simulink model "mdIGBTControlledCurrentSource"  (Simulink 7.3)
settings: Solver=ode45  StartTime=0.0  StopTime=0.5  RelTol=1e-3
libraries: powerlib x14
settings Model: Creator=Think79  LastModifiedBy=Think79

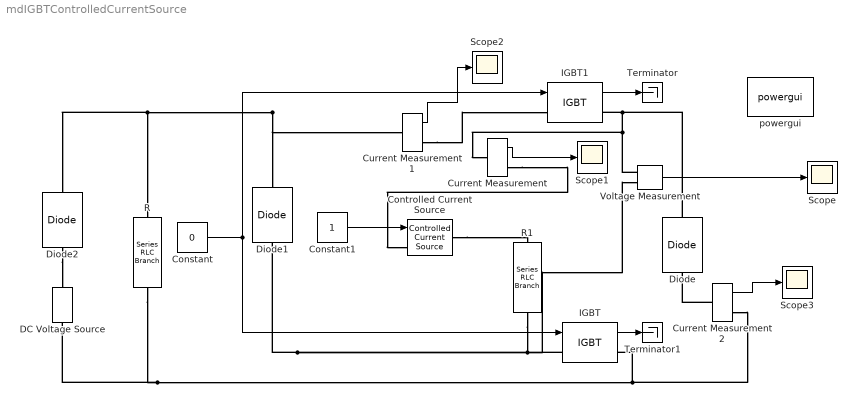
== system mdIGBTControlledCurrentSource ==
  Constant : Constant  Value=0  OutDataType=fixdt(1, 16)  OutScaling=2^0
  Constant1 : Constant  OutDataType=fixdt(1, 16)  OutScaling=2^0
  Controlled Current Source : powerlib/Electrical Sources/Controlled Current Source  DialogController=POWERSYS.PowerSysDialog  SystemSampleTime=-1  Initialize=on  Source_Type=AC  Amplitude=0  Phase=0  Frequency=0  Measurements=None
  Current Measurement : powerlib/Measurements/Current Measurement  DialogController=POWERSYS.PowerSysDialog  SystemSampleTime=-1  PhasorSimulation=off  OutputType=Complex  PSBequivalent=0
  Current Measurement1 : powerlib/Measurements/Current Measurement  DialogController=POWERSYS.PowerSysDialog  SystemSampleTime=-1  PhasorSimulation=off  OutputType=Complex  PSBequivalent=0
  Current Measurement2 : powerlib/Measurements/Current Measurement  DialogController=POWERSYS.PowerSysDialog  SystemSampleTime=-1  PhasorSimulation=off  OutputType=Complex  PSBequivalent=0
  DC Voltage Source : powerlib/Electrical Sources/DC Voltage Source  DialogController=POWERSYS.PowerSysDialog  SystemSampleTime=-1  Amplitude=60  Measurements=None
  Diode : powerlib/Power Electronics/Diode  DialogController=POWERSYS.PowerSysDialog  SystemSampleTime=-1  Ron=0.001  Lon=0  Vf=0.8  IC=0  UseSnubber=off  Rs=500  Cs=250e-9  Measurements=off
  Diode1 : powerlib/Power Electronics/Diode  DialogController=POWERSYS.PowerSysDialog  SystemSampleTime=-1  Ron=0.001  Lon=0  Vf=0.8  IC=0  UseSnubber=off  Rs=500  Cs=250e-9  Measurements=off
  Diode2 : powerlib/Power Electronics/Diode  DialogController=POWERSYS.PowerSysDialog  SystemSampleTime=-1  Ron=0.001  Lon=0  Vf=0.8  IC=0  UseSnubber=off  Rs=500  Cs=250e-9  Measurements=off
  IGBT : powerlib/Power Electronics/IGBT  DialogController=POWERSYS.PowerSysDialog  SystemSampleTime=-1  Ron=0.001  Lon=0  Vf=1  Tf=1e-6  Tt=2e-6  IC=0  Rs=1e5  Cs=inf  Measurements=on
  IGBT1 : powerlib/Power Electronics/IGBT  DialogController=POWERSYS.PowerSysDialog  SystemSampleTime=-1  Ron=0.001  Lon=0  Vf=1  Tf=1e-6  Tt=2e-6  IC=0  Rs=1e5  Cs=inf  Measurements=on
  R : powerlib/Elements/Series RLC Branch  DialogController=POWERSYS.PowerSysDialog  PhysicalDomain=powersysdomain  SubClassName=unknown  LeftPortType=p1  RightPortType=p1  LConnTagsString=__new0  RConnTagsString=__new0  BranchType=R  Resistance=1  Inductance=1.0  SetiL0=off  InitialCurrent=0  Capacitance=1.0  Setx0=off  InitialVoltage=0  Measurements=None
  R1 : powerlib/Elements/Series RLC Branch  DialogController=POWERSYS.PowerSysDialog  PhysicalDomain=powersysdomain  SubClassName=unknown  LeftPortType=p1  RightPortType=p1  LConnTagsString=__new0  RConnTagsString=__new0  BranchType=R  Resistance=0.0261014  Inductance=1.0  SetiL0=off  InitialCurrent=0  Capacitance=1.0  Setx0=off  InitialVoltage=0  Measurements=None
  Scope{,1..3} (4 alike) : Scope
      Scope settings: TimeRange=0.5  YMin=-60  YMax=60
      Scope1 settings: TimeRange=0.5  YMin=-60  YMax=60
      Scope2 settings: TimeRange=0.5  YMin=-60  YMax=60  SaveName=ScopeData2
      Scope3 settings: TimeRange=0.5  YMin=-60  YMax=60  SaveName=ScopeData3
  Terminator : Terminator
  Terminator1 : Terminator
  Voltage Measurement : powerlib/Measurements/Voltage Measurement  DialogController=POWERSYS.PowerSysDialog  SystemSampleTime=-1  PhasorSimulation=off  OutputType=Complex  PSBequivalent=0
  powergui : powerlib/powergui  Priority=1  SystemSampleTime=-1  SimulationMode=Continuous  SampleTime=50e-6  frequency=60  SPID=off  DisableSnubberDevices=off  DisableRonSwitches=off  DisableVfSwitches=off  SwTol=0  Interpol=off  frequencyindice=0  echomessages=off  HookPort=off  DisplayEquations=off  FunctionMessages=off  EnableUseOfTLC=off  x0status=blocks  RestoreLinks=warning  Frange=[0:2:500]  Ylog=off  Xlog=on  ShowGrid=off  save=off  variable=ZData  ZoomFFT=on  StartTime=0.0  cycles=1  DisplayStyle=1  fundamental=60  FreqAxis=off  MaxFrequency=1000  frequencyindicesteady=1  RmsSteady=1  display=off  Ts=0  methode=off
  wires:
  IGBT/1 -> Terminator1/1
  IGBT1/1 -> Terminator/1
  Constant/1 -> IGBT/1, IGBT1/1
  Voltage Measurement/1 -> Scope/1
  Constant1/1 -> Controlled Current Source/1
  Current Measurement/1 -> Scope1/1
  Current Measurement1/1 -> Scope2/1
  Current Measurement2/1 -> Scope3/1
  connections:
  Diode2/LConn1 -- DC Voltage Source/RConn1
  Diode2/RConn1 -- R/LConn1 -- Diode1/RConn1 -- Current Measurement1/LConn1
  Current Measurement/LConn1 -- Voltage Measurement/LConn1 -- Diode/RConn1 -- IGBT1/RConn1
  DC Voltage Source/LConn1 -- R/RConn1 -- IGBT/RConn1 -- Current Measurement2/RConn1
  IGBT/LConn1 -- Diode1/LConn1 -- Voltage Measurement/LConn2 -- R1/RConn1
  Controlled Current Source/RConn1 -- R1/LConn1
  Current Measurement/RConn1 -- Controlled Current Source/LConn1
  Current Measurement1/RConn1 -- IGBT1/LConn1
  Current Measurement2/LConn1 -- Diode/LConn1
